simulink model "Final_activity_sim"  (R2024b)
settings: Solver=VariableStepAuto  StartTime=0.0  StopTime=100  MaxStep=0.001  RelTol=1e-3
undefined symbols (not defined in the file or in its folder): d, D, omega_M, P_INIT_EKF, Q_INIT, r, R_5, T_a, T_c, T_s, Ts, X, x_coords, Y, y_coords, Z_INIT_EKF
libraries: robotlib x4
settings Model: Creator=alber  LastModifiedBy=eugen
settings DebuggingCC: UnderSpecifiedDimensionMsg=warning
settings RTWCC: GPUComputeCapability=3.5

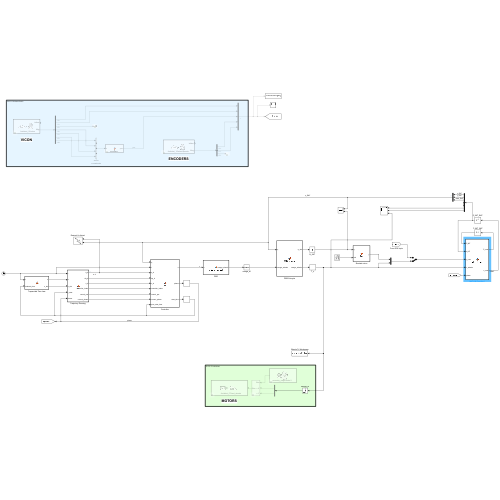
[thumbnail: Simulink's stored preview of the top-level diagram]
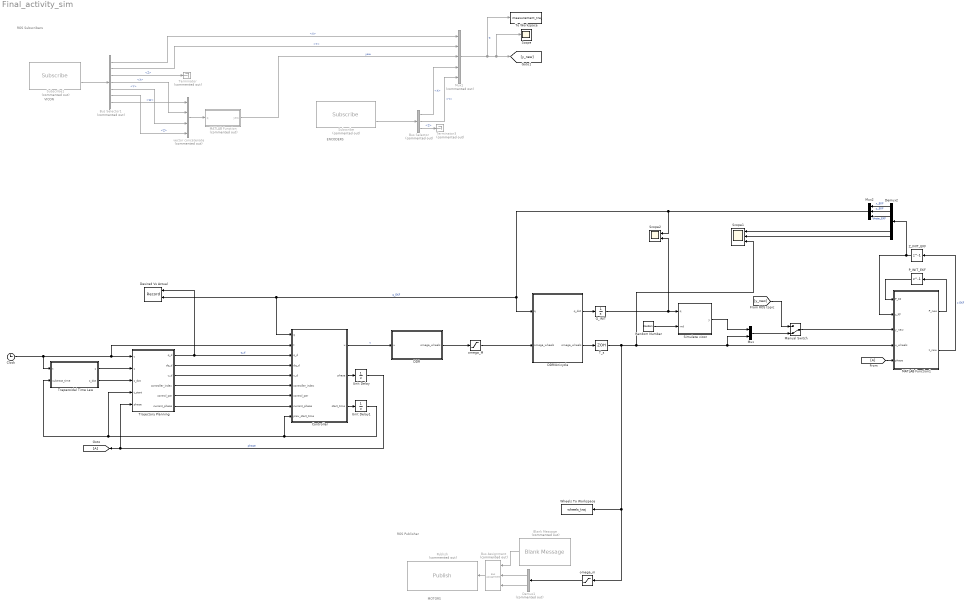
== system Final_activity_sim ==
  note: MOTORS
  note: ROS Publisher
  note: ENCODERS
  note: ROS Subscribers
  note: VICON
  Blank Message : robotlib/Blank Message  Commented=on  messageClass=Message  entityType=geometry_msgs/Vector3  messageType=geometry_msgs/Vector3  SampleTime=Ts  legacyBusStruct=off
      settings: LibrarySourceBlock=roslib/ROS/Blank Message
  Bus Assignment : BusAssignment  Commented=on  AssignedSignals=X,Y
  Bus Selector : BusSelector  Commented=on  OutputSignals=X,Y,Z
  Bus Selector1 : BusSelector  Commented=on  OutputSignals=Pose.Pose.Position.X,Pose.Pose.Position.Y,Pose.Pose.Position.Z,Pose.Pose.Orientation.X,Pose.Pose.Orientation.Y,Pose.Pose.Orientation.Z,Pose.Pose.Orientation.W
  Clock : Clock
  Controller : MATLAB Function  TreatAsAtomicUnit=on
  DDR : MATLAB Function  TreatAsAtomicUnit=on
  DDR/Unicycle : MATLAB Function  TreatAsAtomicUnit=on
  Demux1 : Demux  Commented=on  Outputs=2
  Demux2 : Demux  Outputs=7
  "Desired Vs Actual " : Record  FileSettingsInternal="{\"entries\":[{\"content\":{\"excelSettings\":{\"content\":{},\"type\":\"Streamout.ExcelSettings\"}},\"type\":\"Streamout.FileSettingStorage\",\"uuid\":\"\"}],\"packageUris\":[\"http:\\/\\/schema.mathworks.com\\/mf0\\/streamout_blocks\\/R2020a\"],\"version\":\"1.0\"}"  Layout=[1 1]  SignalsInternal="{\"entries\":[{\"content\":{\"signals\":[{\"content\":{\"blockPath\":[],\"dimensions\":[3,1],\"domain\":\"\",\"hasChildren\":true,\"lineColor\":\"#7e2f8e\",\"lineWidth\":2,\"port\":1,\"sid\":[\"\"],\"signalID\":1,\"signalName\":\"q_d\"},\"type\":\"RecordBlkView.Signal\",\"uuid\":\"\"},{\"content\":{\"blockPath\":[],\"channel\":[1,1],\"dimensions\":[3,1],\"domain\":\"\",\"lineColor\":\"#0072bd\",\"lineWidth\":2,\"parentID\":1,\"port\":1,\"sid\":[\"\"],\"signalID\":2,\"signalName\":\"q_d\"},\"type\":\"RecordBlkView.Signal\",\"uuid\":\"\"},{\"content\":{\"blockPath\":[],\"dimensions\":[3],\"domain\":\"\",\"hasChildren\":true,\"lineColor\":\"#4dbeee\",\"lineWidth\":2,\"port\":2,\"sid\":[\"\"],\"signalID\":3,\"signalName\":\"q_EKF\"},\"type\":\"RecordBlkView.Signal\",\"uuid\":\"\"},{\"content\":{\"blockPath\":[],\"channel\":[1],\"dimensions\":[3],\"domain\":\"\",\"lineColor\":\"#edb120\",\"lineWidth\":2,\"parentID\":3,\"plots\":[ 1 ],\"port\":2,\"sid\":[\"\"],\"signalID\":4,\"signalName\":\"q_EKF\"},\"type\":\"RecordBlkView.Signal\",\"uuid\":\"\"},{\"content\":{\"blockPath\":[],\"channel\":[2,1],\"dimensions\":[3,1],\"domain\":\"\",\"lineColor\":\"#d95319\",\"lineWidth\":2,\"parentID\":1,\"port\":1,\"sid\":[\"\"],\"signalID\":5,\"signalName\":\"q_d\"},\"type\":\"RecordBlkView.Signal\",\"uuid\":\"\"},{\"content\":{\"blockPath\":[],\"channel\":[3,1],\"dimensions\":[3,1],\"domain\":\"\",\"lineColor\":\"#edb120\",\"lineWidth\":2,\"parentID\":1,\"port\":1,\"sid\":[\"\"],\"signalID\":6,\"signalName\":\"q_d\"},\"type\":\"RecordBlkView.Signal\",\"uuid\":\"\"},{\"content\":{\"blockPath\":[],\"channel\":[2],\"dimensions\":[3],\"domain\":\"\",\"lineColor\":\"#139fff\",\"lineWidth\":2,\"parentID\":3,\"plots\":[ 1 ],\"port\":2,\"sid\":[\"\"],\"signalID\":7,\"signalName\":\"q_EKF\"},\"type\":\"RecordBlkView.Signal\",\"uuid\":\"\"},{\"content\":{\"blockPath\":[],\"channel\":[3],\"dimensions\":[3],\"domain\":\"\",\"lineColor\":\"#ff6929\",\"lineWidth\":2,\"parentID\":3,\"port\":2,\"sid\":[\"\"],\"signalID\":8,\"signalName\":\"q_EKF\"},\"type\":\"RecordBlkView.Signal\",\"uuid\":\"\"}]},\"type\":\"RecordBlkView.InputSignals\",\"uuid\":\"\"}],\"packageUris\":[\"http:\\/\\/schema.mathworks.com\\/mf0\\/streamout_blocks\\/R2020a\"],\"version\":\"1.0\"}"  VisualizationBindings="{\"xyplotplugin\":{\"info\":[{\"series\":[{\"bindingParametersList\":[{\"parameter\":\"X-Axis\",\"signalID\":4,\"signalName\":\"q_EKF(1)\"},{\"parameter\":\"Y-Axis\",\"signalID\":7,\"signalName\":\"q_EKF(2)\"}],\"seriesID\":0}],\"subplotID\":1}]}}"  CompatibilityTag=XY
  From : From
  Goto : Goto
  MATLAB Function : MATLAB Function  Commented=on  TreatAsAtomicUnit=on
  MATLAB Function1 : MATLAB Function  TreatAsAtomicUnit=on
  Manual Switch : ManualSwitch  CurrentSetting=0
  Mux : Mux  Inputs=2
  Mux1 : Mux  Commented=on  Inputs=5
  Mux2 : Mux  Inputs=3
  P_INIT_EKF : Delay  DelayLength=1  InitialCondition=P_INIT_EKF  SampleTime=T_s
  Publish : robotlib/Publish  Commented=on  topicSource=Specify your own  topic=/turtlebot_07/cmd_wheels  messageType=geometry_msgs/Vector3  legacyBusStruct=off  messageQueueLength=1
      settings: LibrarySourceBlock=roslib/ROS/Publish
  Q_INIT : Integrator  InitialCondition=Q_INIT
  Random Number : RandomNumber  SampleTime=0.1
  Scope : Scope
  Scope1 : Scope  NumInputPorts=3
  Scope2 : Scope  NumInputPorts=2
  Simulate vicon : MATLAB Function  TreatAsAtomicUnit=on
  Subscribe : robotlib/Subscribe  Commented=on  topicSource=Specify your own  topic=/turtlebot_10/wheelSpeeds  messageType=geometry_msgs/Vector3  SampleTime=-1  legacyBusStruct=off  messageQueueLength=1
      settings: LibrarySourceBlock=roslib/ROS/Subscribe
  Subscribe1 : robotlib/Subscribe  Commented=on  topicSource=Specify your own  topic=/turtlebot_10/odom  messageType=nav_msgs/Odometry  SampleTime=-1  legacyBusStruct=off  messageQueueLength=1
      settings: LibrarySourceBlock=roslib/ROS/Subscribe
  T_s : ZeroOrderHold  SampleTime=T_s
  Terminator : Terminator  Commented=on
  Terminator3 : Terminator  Commented=on
  To Workspace : ToWorkspace  VariableName=measurement_traj  SaveFormat=Timeseries  SampleTime=-1
  Trajectory Planning : MATLAB Function  TreatAsAtomicUnit=on
  Trapezoidal Time Law : MATLAB Function  TreatAsAtomicUnit=on
  Unit Delay : UnitDelay  InitialCondition=1  SampleTime=T_s  HasFrameUpgradeWarning=on
  Unit Delay1 : UnitDelay  InitialCondition=inf  SampleTime=T_s  HasFrameUpgradeWarning=on
  Wheels To Workspace : ToWorkspace  VariableName=wheels_traj  SaveFormat=Timeseries  SampleTime=-1
  Z_INIT_EKF : Delay  DelayLength=1  InitialCondition=Z_INIT_EKF  SampleTime=T_s
  omega_M : Saturate  UpperLimit=omega_M  LowerLimit=-omega_M
  omega_m : Saturate  UpperLimit=omega_M  LowerLimit=-omega_M
  vector concatenate : Concatenate  Commented=on  NumInputs=4
  wires:
  Trajectory Planning/1(q_d) -> Controller/3(q_d), "Desired Vs Actual "/1  "q_d"
  Trajectory Planning/2(dq_d) -> Controller/4(dq_d)
  Trajectory Planning/3(u_d) -> Controller/5(u_d)
  Trajectory Planning/4(controller_index) -> Controller/6(controller_index)
  Trajectory Planning/5(control_par) -> Controller/7(control_par)
  MATLAB Function1/2(z_new) -> Z_INIT_EKF/1  "z EKF"
  P_INIT_EKF/1 -> MATLAB Function1/1(P_KF)
  MATLAB Function1/1(P_new) -> P_INIT_EKF/1
  DDR/1(omega_wheels) -> omega_M/1
  Controller/1(u) -> DDR/1(u)  "u"
  Clock/1 -> Trajectory Planning/1(t), Controller/2(t), Trapezoidal Time Law/1(t)
  Unit Delay/1 -> Goto/1, Trajectory Planning/5(phase)  "phase"
  Trapezoidal Time Law/1(s) -> Trajectory Planning/2(s)
  Random Number/1 -> Simulate vicon/2(rnd)
  Simulate vicon/1(y) -> Mux/1
  Q_INIT/1 -> Scope2/2, Simulate vicon/1(q)
  Trajectory Planning/6(current_phase) -> Controller/8(current_phase)
  Controller/3(start_time) -> Unit Delay1/1
  Unit Delay1/1 -> Trapezoidal Time Law/2(subtract_time), Trajectory Planning/4(t_start), Controller/9(prev_start_time)
  Trapezoidal Time Law/2(s_dot) -> Trajectory Planning/3(s_dot)
  DDR/Unicycle/1(q_dot) -> Q_INIT/1
  omega_M/1 -> DDR/Unicycle/2("omega_wheels ")
  DDR/Unicycle/2(omega_wheels) -> T_s/1
  Controller/2(phase) -> Unit Delay/1
  Mux2/1 -> DDR/Unicycle/1(q), Controller/1(q), "Desired Vs Actual "/2, Scope2/1  "q_EKF"
  Z_INIT_EKF/1 -> MATLAB Function1/2(z_KF), Demux2/1
  Demux2/2 -> Mux2/2  "y_EKF"
  Demux2/3 -> Mux2/3  "theta_EKF"
  Demux2/1 -> Mux2/1  "x_EKF"
  Blank Message/1 -> Bus Assignment/1
  Demux1/2 -> Bus Assignment/3
  Bus Assignment/1 -> Publish/1
  Demux1/1 -> Bus Assignment/2
  omega_m/1 -> Demux1/1
  T_s/1 -> Scope1/3, Mux/2, MATLAB Function1/4(u_wheels), omega_m/1, Wheels To Workspace/1
  From/1 -> MATLAB Function1/5(phase)
  Subscribe1/2 -> Bus Selector1/1
  Bus Selector1/7 -> vector concatenate/1  "<W>"
  Mux1/1 -> To Workspace/1, [y_new], Scope/1  "q"
  Bus Selector1/2 -> Mux1/2  "<Y>"
  Bus Selector/1 -> Mux1/4  "<X>"
  Bus Selector1/5 -> vector concatenate/3  "<Y>"
  Bus Selector1/6 -> vector concatenate/4  "<Z>"
  Bus Selector/2 -> Mux1/5  "<Y>"
  Subscribe/2 -> Bus Selector/1
  vector concatenate/1 -> MATLAB Function/1(q)
  Bus Selector1/3 -> Terminator/1  "<Z>"
  MATLAB Function/1(yaw) -> Mux1/3  "yaw"
  Bus Selector/3 -> Terminator3/1  "<Z>"
  Bus Selector1/4 -> vector concatenate/2  "<X>"
  Bus Selector1/1 -> Mux1/1  "<X>"
  Manual Switch/1 -> MATLAB Function1/3(y_new)
  [y_new] -> Manual Switch/1
  Mux/1 -> Manual Switch/2
  Demux2/7 -> Scope1/2
  Demux2/6 -> Scope1/1

== matlab function Final_activity_sim/DDR ==
  data: u input; omega_wheels output; r parameter; d parameter
function omega_wheels = kin2omegawheels(u, r, d)
omega_l = u(1)/r-d/(2*r)*u(2);
omega_r = u(1)/r+d/(2*r)*u(2);
omega_wheels = [omega_l;omega_r];

== matlab function Final_activity_sim/DDR//Unicycle ==
  data: q input; omega_wheels input; q_dot output; omega_wheels output; d parameter; r parameter
function [q_dot,  omega_wheels]  = DDR_Unicycle(q, omega_wheels, d, r)
omega_wheels = omega_wheels;
u = [r*(omega_wheels(1)+omega_wheels(2))/2; r*(-omega_wheels(1)+omega_wheels(2))/d];

q_dot = [cos(q(3))*u(1);
    sin(q(3))*u(1);
    u(2)];

end

== matlab function Final_activity_sim/Trapezoidal Time Law ==
  data: s output; t input; T_a parameter; s_dot output; T_c parameter; subtract_time input
function [s,s_dot]=fcn(t, T_a, T_c, subtract_time)

    v_c = 1 / (T_a + T_c);
    a = v_c / T_a;
    
    % we get the start time of the trajectory tracking 
    t = t - subtract_time;

    if(t < 0)
        s_dot = 0;
        s = 0;
    elseif(t > 2*T_a+T_c)
        s_dot = 0;
        s = 1;
    elseif(t > T_a+T_c)
        s_dot = v_c - a * (t - T_a - T_c);
        s = (a * T_a^2)/2 + v_c * (t - T_a - T_c) + v_c * (T_c) - (a * (t - T_c - T_a)^2)/2;
    elseif(t > T_a)
        s_dot = v_c; 
        s = (a * T_a^2)/2 + v_c * (t - T_a);
    else 
        s_dot = a * t;
        s = (a * t^2)/2;
    end
    
end

== matlab function Final_activity_sim/MATLAB Function ==
  data: q input; yaw output
function yaw = quat2yaw(q)

% normalize to avoid issues
q = q / norm(q);

w = q(1);
x = q(2);
y = q(3);
z = q(4);

% rotation around Z axis
yaw = atan2(2*(w*z + x*y), 1 - 2*(y^2 + z^2));

end

== matlab function Final_activity_sim/Simulate vicon ==
  data: q input; rnd input; y output; x_coords parameter; y_coords parameter
function y = fcn(q, rnd, x_coords, y_coords)

if (q(1) > x_coords(5) && q(1) < x_coords(6) && q(2) > y_coords(1) && q(2) < y_coords(6))

    % red area
    y = [0;0;0];

elseif (q(1) > x_coords(7) && q(1) < x_coords(11) && q(2) > y_coords(1) && q(2) < y_coords(8))

    % orange area 
    if(rnd < 0.1)
        y = q;
    else 
        y = [0;0;0];
    end 
    
else 
    
    % white area
    y = q;

end

%bypass
%y = q;

== matlab function Final_activity_sim/Trajectory Planning ==
  data: x_coords parameter; y_coords parameter; t input; s input; s_dot input; t_start input; phase input; q_d output; dq_d output; u_d output; controller_index output; control_par output; current_phase output
function [q_d,dq_d,u_d,controller_index,control_par,current_phase] = fcn(x_coords,y_coords,t, s, s_dot,t_start, phase)

% regulation
if phase == 1

    controller_index = 1;

    q_d = [x_coords(2);y_coords(2);0];
    dq_d = [0;0;0];
    u_d = [0;0];
    control_par = [0.2,0.5,1];
    current_phase = 1;

    % Cartesian polinomials
elseif phase == 2

    controller_index = 2;

    q_i = [x_coords(2), y_coords(2), 0];
    q_f = [x_coords(8), y_coords(4), 0];
    k_i = 5;
    k_f = 5;
    k_sign = sign(k_i);

    y = [0,0,0,0;0,0,0,0];
    y(1,1) = q_f(1);
    y(1,2) = q_i(1);
    y(1,3) = k_f * cos(q_f(3)) - 3 * q_f(1);
    y(1,4) = k_i * cos(q_i(3)) + 3 * q_i(1);

    y(2,1) = q_f(2);
    y(2,2) = q_i(2);
    y(2,3) = k_f * sin(q_f(3)) - 3 * q_f(2);
    y(2,4) = k_i * sin(q_i(3)) + 3 * q_i(2);


    x_exp = y(1,1) * s^3 - y(1,2) * (s - 1)^3 + y(1,3) * s^2 * (s - 1) + y(1,4) * s * (s - 1)^2;
    y_exp = y(2,1) * s^3 - y(2,2) * (s - 1)^3 + y(2,3) * s^2 * (s - 1) + y(2,4) * s * (s - 1)^2;

    x_dot = 3 * y(1,1) * s^2 - 3 * y(1,2) * (s-1)^2 + 2 * y(1,3) * s * (s-1) + y(1,3) * s^2 + y(1,4) * (s-1)^2 + 2 * y(1,4) * s * (s-1);
    y_dot = 3 * y(2,1) * s^2 - 3 * y(2,2) * (s-1)^2 + 2 * y(2,3) * s * (s-1) + y(2,3) * s^2 + y(2,4) * (s-1)^2 + 2 * y(2,4) * s * (s-1);
    x_dotdot = 6 * y(1,1) * s - 6 * y(1,2) * (s-1) + 2 * y(1,3) * s + 2 * y(1,3) * (s-1) + 2 * s * y(1,3) + 2 * y(1,4) * (s-1) + 2 * y(1,4) * s + 2 * y(1,4) * (s-1);
    y_dotdot = 6 * y(2,1) * s - 6 * y(2,2) * (s-1) + 2 * y(2,3) * s + 2 * y(2,3) * (s-1) + 2 * s * y(2,3) + 2 * y(2,4) * (s-1) + 2 * y(2,4) * s + 2 * y(2,4) * (s-1);


    if(k_sign == 1)
        v = sqrt((x_dot)^2 + (y_dot)^2) * s_dot;
        theta_exp = atan2(y_dot,x_dot) + pi;
    else
        v = - sqrt((x_dot)^2 + (y_dot)^2) * s_dot;
        theta_exp = atan2(y_dot,x_dot);
    end

    q_d = [x_exp; y_exp; wrapToPi(theta_exp)];

    w = (((x_dot) * (y_dotdot) - (y_dot) * (x_dotdot)) / ((x_dot)^2 + (y_dot)^2)) * s_dot;

    u_d = [v;w];

    x_prime = x_dot * s_dot;
    y_prime = y_dot * s_dot;

    dq_d = [x_prime; y_prime; w];

    control_par = [0.1,0.1,0.01];

    current_phase = 2;

    % circle and a half
elseif phase == 3

    controller_index = 2;
    R = 0.8;
    T_trj = 40;
    x_center = 2.29;
    y_center = 0.1;
    omega = 2 * pi / T_trj;

    theta_offset = deg2rad(210);
 
    theta = 1.5 * omega * (t - t_start) + theta_offset;

    x_d = x_center + R * cos(theta);
    dx_d = -R * 1.5 * omega * sin(theta);
    ddx_d = -R * (1.5 * omega)^2 * cos(theta);

    y_d = y_center + R * sin(theta);
    dy_d = R * 1.5 * omega * cos(theta);
    ddy_d = -R * (1.5 * omega)^2 * sin(theta);

    theta_d = atan2(dy_d, dx_d);
    dtheta_d = (dx_d * ddy_d - dy_d * ddx_d) / (dx_d^2 + dy_d^2);

    q_d = [x_d; y_d; theta_d];
    dq_d = [dx_d; dy_d; dtheta_d];
    u_d = [sqrt(dx_d^2 + dy_d^2); dtheta_d];

    control_par = [0.1, 0.1, 0.01];
    current_phase = 3;


else 

    controller_index = 1;

    q_d = [x_coords(2);y_coords(2);0];
    dq_d = [0;0;0];
    u_d = [0;0];
    control_par = [0.2,0.5,1];
    current_phase = 1;

end



end

== matlab function Final_activity_sim/Controller ==
  data: u output size=[2,1]; q input; t input; q_d input; dq_d input; u_d input; controller_index input; control_par input; x_coords parameter; y_coords parameter; current_phase input; prev_start_time input; phase output size=1; start_time output size=1
function [u,phase,start_time]  = fcn(q, t, q_d, dq_d, u_d, controller_index, control_par, x_coords, y_coords, current_phase,prev_start_time)

if controller_index == 1
    % posture regulation
    % transform q
    % compute pointing error
    phase = 1;
    start_time = prev_start_time;

    R = [cos(q_d(3)), sin(q_d(3)), 0;
        -sin(q_d(3)), cos(q_d(3)), 0;
        0, 0, 1];
    p_prime = R*(q - q_d);
    rho = sqrt(p_prime(1)^2 + p_prime(2)^2);
    gamma = wrapToPi(atan2(p_prime(2), p_prime(1))+pi-p_prime(3));
    delta = p_prime(3) + gamma;
    if abs(gamma)<1e-4
        u = [control_par(1)*rho*cos(gamma); control_par(2)*gamma + control_par(1)*cos(gamma)*(gamma + control_par(3)*delta)];
    else
        u = [control_par(1)*rho*cos(gamma); control_par(2)*gamma + control_par(1)*sin(gamma)*cos(gamma)*(gamma + control_par(3)*delta)/gamma];
    end

    % switch to next phase feedback linearization
    if abs(q(1) - x_coords(2)) <= 0.05 && abs(q(2) - y_coords(2)) <= 0.05
        phase = 2;
        start_time = t;
    end

else %if controller_index == 2

    start_time = prev_start_time;

    % feedback linearization
    %control_par = [k1, k2,b];
    k1=control_par(1);
    k2=control_par(2);
    b=control_par(3);

    %evaluation b point
    Xb=q(1)+b*cos(q(3));
    Yb=q(2)+b*sin(q(3));

    %evaluation b point desired
    Xb_d=q_d(1)+b*cos(q_d(3));
    Yb_d=q_d(2)+b*sin(q_d(3));

    %evaluation derivatives b point desired
    dXb_d=dq_d(1)-b*sin(q_d(3))*dq_d(3);
    dYb_d=dq_d(2)+b*cos(q_d(3))*dq_d(3);

    %matrix b poit to point
    T_inv=[ cos(q(3)),      sin(q(3));
            -sin(q(3))/b,   cos(q(3))/b];

    %evaluation of controll law
    u = T_inv*[ dXb_d+k1*(Xb_d-Xb);
                dYb_d+k2*(Yb_d-Yb)];


    if  current_phase == 2
        % switch to next phase, circle around obstacle at [1.45; -0.3]
        if abs(q(1) - x_coords(8)) <= 0.1 && abs(q(2) - y_coords(4)) <= 0.1
            phase = 3;
            start_time = t;
        else
            phase = 2;
        end
    else
        phase = 3;
    end

end

end

== matlab function Final_activity_sim/MATLAB Function1 ==
  data: P_KF input; P_new output; z_KF input; y_new input; z_new output; u_wheels input; D parameter; R_5 parameter; T_s parameter; r parameter; d parameter; phase input
function [P_new, z_new] = EKF_filtering(P_KF, z_KF, y_new, u_wheels, D, R_5, T_s, r, d, phase)

% z_KF = [x_EKF, y_EKF, theta_EKF, delta_phi_L_EKF, delta_phi_R_EKF, omega_L_EKF, omega_R_EKF]

v_k = r * (z_KF(6) + z_KF(7))/2;
w_k = r * (z_KF(7) - z_KF(6))/d;
theta_mean = z_KF(3) + (w_k * T_s)/2;

F_k = [1, 0, -T_s * v_k * sin(theta_mean), 0, 0, T_s * r * cos(theta_mean)/2 + (T_s)^2 * r * v_k * sin(theta_mean)/(2*d), T_s * r * cos(theta_mean)/2 - (T_s)^2 * r * v_k * sin(theta_mean)/(2*d);
       0, 1,  T_s * v_k * cos(theta_mean), 0, 0, T_s * r * sin(theta_mean)/2 - (T_s)^2 * r * v_k * cos(theta_mean)/(2*d), T_s * r * sin(theta_mean)/2 + (T_s)^2 * r * v_k * cos(theta_mean)/(2*d);
       0, 0, 1, 0, 0, (-T_s*r)/d, (T_s*r)/d;
       0, 0, 0, 0, 0, T_s, 0;
       0, 0, 0, 0, 0, 0, T_s;
       0, 0, 0, 0, 0, 0, 0;
       0, 0, 0, 0, 0, 0, 0];

%% Prediction part

z_pred = [z_KF(1)+(T_s*r*(z_KF(6)+z_KF(7))/2)*cos(theta_mean + (T_s*r*(z_KF(6)+z_KF(7)))/(2*d)); 
          z_KF(2)+(T_s*r*(z_KF(6)+z_KF(7))/2)*sin(theta_mean + (T_s*r*(z_KF(7)-z_KF(6)))/(2*d));
          theta_mean + (T_s*r*(z_KF(7)-z_KF(6))/(2*d));
          T_s*z_KF(6);
          T_s*z_KF(7);
          u_wheels(1);
          u_wheels(2)];
z_pred(3) = wrapToPi(z_pred(3));
P_pred = F_k * P_KF * F_k' + D;


if (phase == 3)
    %% Encoders + GPS + LiDAR
    y_new_1 = y_new(1:5);

    H = [1, 0, 0, 0, 0, 0, 0;
        0, 1, 0, 0, 0, 0, 0;
        0, 0, 1, 0, 0, 0, 0;
        0, 0, 0, 0, 0, 1, 0;
        0, 0, 0, 0, 0, 0, 1];

    e = y_new_1 - H * z_pred;
    K = P_pred * H' / (H * P_pred * H' + R_5);

    e(3) = wrapToPi(e(3));

    z_new = z_pred + K * e;
    P_new = P_pred - K * H * P_pred;
else
    %% Encoders + GPS
    y_new_1 = y_new(1:5);

    H = [1, 0, 0, 0, 0, 0, 0;
        0, 1, 0, 0, 0, 0, 0;
        0, 0, 1, 0, 0, 0, 0;
        0, 0, 0, 0, 0, 1, 0;
        0, 0, 0, 0, 0, 0, 1];

    e = y_new_1 - H * z_pred;
    K = P_pred * H' / (H * P_pred * H' + R_5);

    e(3) = wrapToPi(e(3));

    z_new = z_pred + K * e;
    P_new = P_pred - K * H * P_pred;

end
